simulink library "GAS"  (Simulink 8.5)
settings: Solver=ode45  StartTime=0.0  StopTime=10.0  RelTol=1e-3
undefined symbols (not defined in the file): COILOUTF, SIXOSEM_F_COILOUTF_MASTER, SIXOSEM_F_STAGE_MASTER
libraries: cdsEpicsOut x14, cdsFiltCtrl x4, cdsFilt x4, cdsTP x4, cdsEpicsIn x2, cdsEpicsBinIn x1, cdsFunctionCall x1, VIS_LIB x1
settings Model: Creator=controls  LastModifiedBy=controls

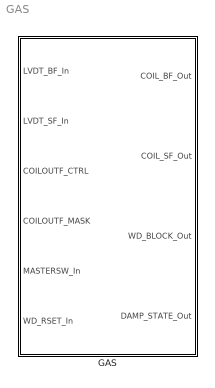
== system GAS ==
  GAS : Subsystem  Description=SIXOSEMSTAGE_FACE_MASTER  AncestorBlock=SIXOSEM_F_STAGE_MASTER/SIXOSEM_F_STAGE_MASTER

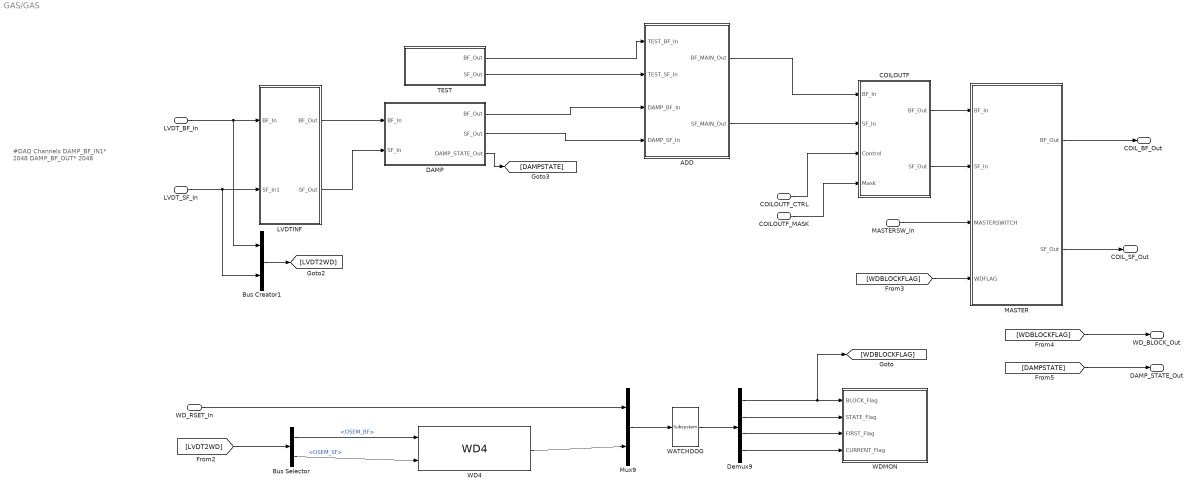
== system GAS/GAS ==
  note: #DAQ Channels
      | DAMP_BF_IN1* 2048
      | DAMP_BF_OUT* 2048
  LVDT_BF_In : Inport
  LVDT_SF_In : Inport  Port=2
  COILOUTF_CTRL : Inport  Port=3
  COILOUTF_MASK : Inport  Port=4
  MASTERSW_In : Inport  Port=5
  WD_RSET_In : Inport  Port=6
  ADD : Subsystem
  Bus Creator1 : BusCreator  Inputs='OSEM_BF','OSEM_SF'
  Bus Selector : BusSelector  OutputSignals=OSEM_BF,OSEM_SF
  COILOUTF : Subsystem  AncestorBlock=SIXOSEM_F_COILOUTF_MASTER/COILOUTF
  DAMP : Subsystem
  Demux9 : Demux
  LVDTINF : Subsystem
  MASTER : Subsystem
  Mux9 : Mux  Inputs=2
  TEST : Subsystem  AncestorBlock=SIXOSEM_F_STAGE_MASTER/SIXOSEM_F_STAGE_MASTER/TEST
  WATCHDOG : cdsFunctionCall/Subsystem  Tag=cdsFunctionCall  Description=inline OSEMWATCHDOG /opt/rtcds/userapps/release/vis/common/src/WATCHDOG.c
      settings: AttributesFormatString=%<Tag>\n%<Description>
  WD4 : VIS_LIB/WD4
  WDMON : Subsystem
  COIL_BF_Out : Outport
  COIL_SF_Out : Outport  Port=2
  WD_BLOCK_Out : Outport  Port=3
  DAMP_STATE_Out : Outport  Port=4
  wires:
  Bus Selector/1 -> WD4/1  "<OSEM_BF>"
  COILOUTF/1(BF_Out) -> MASTER/1(BF_In)
  ADD/1(BF_MAIN_Out) -> COILOUTF/1(BF_In)
  TEST/1(BF_Out) -> ADD/1(TEST_BF_In)
  LVDTINF/1(BF_Out) -> DAMP/1(BF_In)
  WATCHDOG/1 -> Demux9/1
  Mux9/1 -> WATCHDOG/1
  Demux9/4 -> WDMON/4(CURRENT_Flag)
  Demux9/3 -> WDMON/3(FIRST_Flag)
  Demux9/2 -> WDMON/2(STATE_Flag)
  Demux9/1 -> WDMON/1(BLOCK_Flag), [WDBLOCKFLAG]
  MASTER/1(BF_Out) -> COIL_BF_Out/1
  [LVDT2WD] -> Bus Selector/1
  Bus Creator1/1 -> [LVDT2WD]
  LVDT_BF_In/1 -> Bus Creator1/1, LVDTINF/1(BF_In)
  [WDBLOCKFLAG] -> MASTER/4(WDFLAG)
  [WDBLOCKFLAG] -> WD_BLOCK_Out/1
  DAMP/3(DAMP_STATE_Out) -> [DAMPSTATE]
  [DAMPSTATE] -> DAMP_STATE_Out/1
  MASTERSW_In/1 -> MASTER/3(MASTERSWITCH)
  COILOUTF_MASK/1 -> COILOUTF/4(Mask)
  COILOUTF_CTRL/1 -> COILOUTF/3(Control)
  WD4/1 -> Mux9/2
  WD_RSET_In/1 -> Mux9/1
  DAMP/1(BF_Out) -> ADD/3(DAMP_BF_In)
  LVDT_SF_In/1 -> Bus Creator1/2, LVDTINF/2(SF_In1)
  LVDTINF/2(SF_Out) -> DAMP/2(SF_In)
  TEST/2(SF_Out) -> ADD/2(TEST_SF_In)
  DAMP/2(SF_Out) -> ADD/4(DAMP_SF_In)
  ADD/2(SF_MAIN_Out) -> COILOUTF/2(SF_In)
  COILOUTF/2(SF_Out) -> MASTER/2(SF_In)
  MASTER/2(SF_Out) -> COIL_SF_Out/1
  Bus Selector/2 -> WD4/2  "<OSEM_SF>"

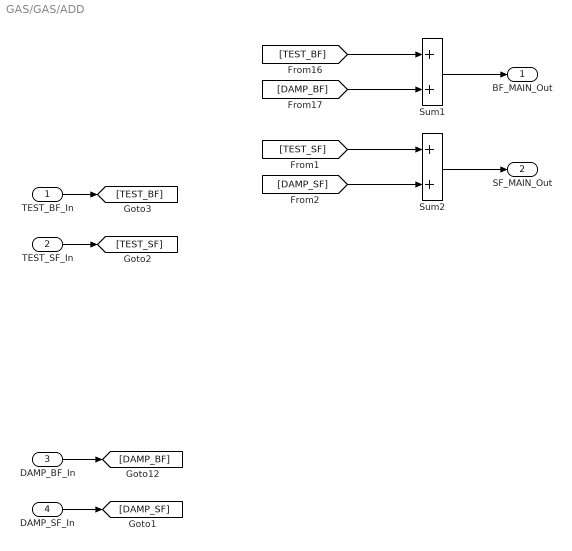
== system GAS/GAS/ADD ==
  TEST_BF_In : Inport
  TEST_SF_In : Inport  Port=2
  DAMP_BF_In : Inport  Port=3
  DAMP_SF_In : Inport  Port=4
  Sum1 : Sum
  Sum2 : Sum
  BF_MAIN_Out : Outport
  SF_MAIN_Out : Outport  Port=2
  wires:
  Sum1/1 -> BF_MAIN_Out/1
  TEST_BF_In/1 -> [TEST_BF]
  DAMP_BF_In/1 -> [DAMP_BF]
  [TEST_BF] -> Sum1/1
  [DAMP_BF] -> Sum1/2
  TEST_SF_In/1 -> [TEST_SF]
  DAMP_SF_In/1 -> [DAMP_SF]
  Sum2/1 -> SF_MAIN_Out/1
  [TEST_SF] -> Sum2/1
  [DAMP_SF] -> Sum2/2

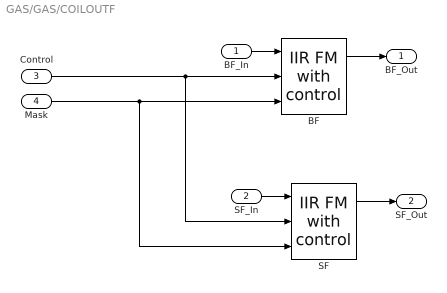
== system GAS/GAS/COILOUTF ==
  BF_In : Inport
  SF_In : Inport  Port=2
  Control : Inport  Port=3
  Mask : Inport  Port=4
  BF : cdsFiltCtrl/IIR FM with control  Tag=cdsFiltCtrl  Description=|
      | cdsFiltCntrl is the standard IIR filter module (exactly the same as cdsFilt) but with added control data output 'Ctrl'. Filter module digital signal output appears on the first output, which is called 'Val'. 'Ctrl' output has a bit pattern encoding the state of filter's on/off switches (FM1 through FM10). The bit values are:
      |                                                                                                                                                                                                                                                                                                                                       
      | module 	hex	dec                                                                                                                                                                                                                                                                                                                       
      | -----------------------                                                                                                                                                                                                                                                                                                               
      | FM1	0x20                    32                                                                                                                                                                                                                                                                                                        
      | FM2	0x80                     128                                                                                                                                                                                                                                                                                                      
      | FM3	0x200                   512                                                                                                                                                                                                                                                                                                       
      | FM4	0x800                   2048                                                                                                                                                                                                                                                                                                      
      | FM5	0x2000                 8192                                                                                                                                                                                                                                                                                                       
      | FM6	0x8000                 32768                                                                                                                                                                                                                                                                                                      
      | FM7	0x20000                131072                                                                                                                                                                                                                                                                                                     
      | FM8	0x80000                 524288                                                                                                                                                                                                                                                                                                    
      | FM9	0x200000               2097152                                                                                                                                                                                                                                                                                                    
      | FM10	0x800000               8388608                                                                                                                                                                                                                                                                                                   
      |                                                                                                                                                                                                                                                                                                                                       
      | This bit data can be used to drive some other switches or it can be output using a binary I/O module.
      settings: AttributesFormatString=%<Tag>
  SF : cdsFiltCtrl/IIR FM with control  Tag=cdsFiltCtrl  Description=|
      | cdsFiltCntrl is the standard IIR filter module (exactly the same as cdsFilt) but with added control data output 'Ctrl'. Filter module digital signal output appears on the first output, which is called 'Val'. 'Ctrl' output has a bit pattern encoding the state of filter's on/off switches (FM1 through FM10). The bit values are:
      |                                                                                                                                                                                                                                                                                                                                       
      | module 	hex	dec                                                                                                                                                                                                                                                                                                                       
      | -----------------------                                                                                                                                                                                                                                                                                                               
      | FM1	0x20                    32                                                                                                                                                                                                                                                                                                        
      | FM2	0x80                     128                                                                                                                                                                                                                                                                                                      
      | FM3	0x200                   512                                                                                                                                                                                                                                                                                                       
      | FM4	0x800                   2048                                                                                                                                                                                                                                                                                                      
      | FM5	0x2000                 8192                                                                                                                                                                                                                                                                                                       
      | FM6	0x8000                 32768                                                                                                                                                                                                                                                                                                      
      | FM7	0x20000                131072                                                                                                                                                                                                                                                                                                     
      | FM8	0x80000                 524288                                                                                                                                                                                                                                                                                                    
      | FM9	0x200000               2097152                                                                                                                                                                                                                                                                                                    
      | FM10	0x800000               8388608                                                                                                                                                                                                                                                                                                   
      |                                                                                                                                                                                                                                                                                                                                       
      | This bit data can be used to drive some other switches or it can be output using a binary I/O module.
      settings: AttributesFormatString=%<Tag>
  BF_Out : Outport
  SF_Out : Outport  Port=2
  wires:
  BF_In/1 -> BF/1
  BF/1 -> BF_Out/1
  Control/1 -> SF/2, BF/2
  Mask/1 -> SF/3, BF/3
  SF_In/1 -> SF/1
  SF/1 -> SF_Out/1

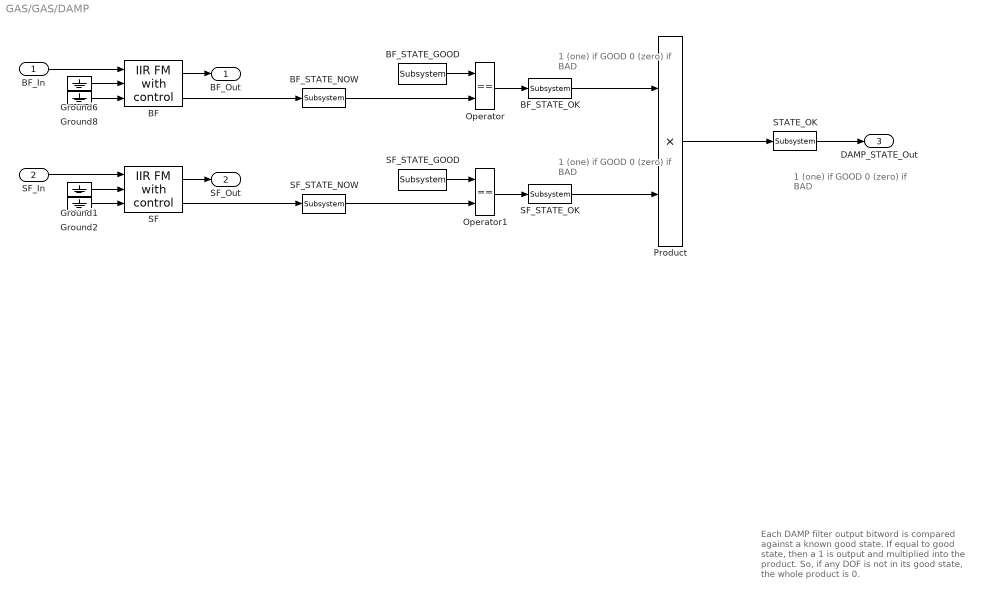
== system GAS/GAS/DAMP ==
  note: Each DAMP filter output bitword is
      | compared against a known good state.
      | If equal to good state, then a 1 is output
      | and multiplied into the product. So, if any DOF
      | is not in its good state, the whole product is 0.
  note: 1 (one) if GOOD
      | 0 (zero) if BAD
  note: 1 (one) if GOOD
      | 0 (zero) if BAD
  note: 1 (one) if GOOD
      | 0 (zero) if BAD
  BF_In : Inport
  SF_In : Inport  Port=2
  BF : cdsFiltCtrl/IIR FM with control  Tag=cdsFiltCtrl  Description=|
      | cdsFiltCntrl is the standard IIR filter module (exactly the same as cdsFilt) but with added control data output 'Ctrl'. Filter module digital signal output appears on the first output, which is called 'Val'. 'Ctrl' output has a bit pattern encoding the state of filter's on/off switches (FM1 through FM10). The bit values are:
      |                                                                                                                                                                                                                                                                                                                                       
      | module 	hex	dec                                                                                                                                                                                                                                                                                                                       
      | -----------------------                                                                                                                                                                                                                                                                                                               
      | FM1	0x20                    32                                                                                                                                                                                                                                                                                                        
      | FM2	0x80                     128                                                                                                                                                                                                                                                                                                      
      | FM3	0x200                   512                                                                                                                                                                                                                                                                                                       
      | FM4	0x800                   2048                                                                                                                                                                                                                                                                                                      
      | FM5	0x2000                 8192                                                                                                                                                                                                                                                                                                       
      | FM6	0x8000                 32768                                                                                                                                                                                                                                                                                                      
      | FM7	0x20000                131072                                                                                                                                                                                                                                                                                                     
      | FM8	0x80000                 524288                                                                                                                                                                                                                                                                                                    
      | FM9	0x200000               2097152                                                                                                                                                                                                                                                                                                    
      | FM10	0x800000               8388608                                                                                                                                                                                                                                                                                                   
      |                                                                                                                                                                                                                                                                                                                                       
      | This bit data can be used to drive some other switches or it can be output using a binary I/O module.
      settings: AttributesFormatString=%<Tag>
  BF_STATE_GOOD : cdsEpicsIn/Subsystem  Tag=cdsEpicsIn  Description=|
      | Purpose:                                                                              
      | Create an EPICS input channel connection to the FE realtime controls.                 
      |                                                                                       
      | Operation:                                                                            
      | Outputs value from an EPICS ai record. Value is floating point with a precision of 3..
      |                                                                                       
      | Usage:                                                                                
      | Name the part with the desired EPICS channel name.
      settings: AttributesFormatString=%<Tag>
  BF_STATE_NOW : cdsEpicsOut/Subsystem  Tag=cdsEpicsOutput  Description=|
      | Purpose:                                          
      | Output a FE signal to an EPICS channel.           
      |                                                   
      | Operation:                                        
      | Takes input value and passes it to EPICS record.  
      |                                                   
      | Usage:                                            
      | Name the part with the desired EPICS rrecord name.
      settings: AttributesFormatString=%<Tag>
  BF_STATE_OK : cdsEpicsOut/Subsystem  Tag=cdsEpicsOutput  Description=|
      | Purpose:                                          
      | Output a FE signal to an EPICS channel.           
      |                                                   
      | Operation:                                        
      | Takes input value and passes it to EPICS record.  
      |                                                   
      | Usage:                                            
      | Name the part with the desired EPICS rrecord name.
      settings: AttributesFormatString=%<Tag>
  Ground{1..2,6,8} (4 alike) : Ground
  Operator : RelationalOperator  Operator===  OutDataTypeStr=boolean
  Operator1 : RelationalOperator  Operator===  OutDataTypeStr=boolean
  Product : Product  RndMeth=Zero
  SF : cdsFiltCtrl/IIR FM with control  Tag=cdsFiltCtrl  Description=|
      | cdsFiltCntrl is the standard IIR filter module (exactly the same as cdsFilt) but with added control data output 'Ctrl'. Filter module digital signal output appears on the first output, which is called 'Val'. 'Ctrl' output has a bit pattern encoding the state of filter's on/off switches (FM1 through FM10). The bit values are:
      |                                                                                                                                                                                                                                                                                                                                       
      | module 	hex	dec                                                                                                                                                                                                                                                                                                                       
      | -----------------------                                                                                                                                                                                                                                                                                                               
      | FM1	0x20                    32                                                                                                                                                                                                                                                                                                        
      | FM2	0x80                     128                                                                                                                                                                                                                                                                                                      
      | FM3	0x200                   512                                                                                                                                                                                                                                                                                                       
      | FM4	0x800                   2048                                                                                                                                                                                                                                                                                                      
      | FM5	0x2000                 8192                                                                                                                                                                                                                                                                                                       
      | FM6	0x8000                 32768                                                                                                                                                                                                                                                                                                      
      | FM7	0x20000                131072                                                                                                                                                                                                                                                                                                     
      | FM8	0x80000                 524288                                                                                                                                                                                                                                                                                                    
      | FM9	0x200000               2097152                                                                                                                                                                                                                                                                                                    
      | FM10	0x800000               8388608                                                                                                                                                                                                                                                                                                   
      |                                                                                                                                                                                                                                                                                                                                       
      | This bit data can be used to drive some other switches or it can be output using a binary I/O module.
      settings: AttributesFormatString=%<Tag>
  SF_STATE_GOOD : cdsEpicsIn/Subsystem  Tag=cdsEpicsIn  Description=|
      | Purpose:                                                                              
      | Create an EPICS input channel connection to the FE realtime controls.                 
      |                                                                                       
      | Operation:                                                                            
      | Outputs value from an EPICS ai record. Value is floating point with a precision of 3..
      |                                                                                       
      | Usage:                                                                                
      | Name the part with the desired EPICS channel name.
      settings: AttributesFormatString=%<Tag>
  SF_STATE_NOW : cdsEpicsOut/Subsystem  Tag=cdsEpicsOutput  Description=|
      | Purpose:                                          
      | Output a FE signal to an EPICS channel.           
      |                                                   
      | Operation:                                        
      | Takes input value and passes it to EPICS record.  
      |                                                   
      | Usage:                                            
      | Name the part with the desired EPICS rrecord name.
      settings: AttributesFormatString=%<Tag>
  SF_STATE_OK : cdsEpicsOut/Subsystem  Tag=cdsEpicsOutput  Description=|
      | Purpose:                                          
      | Output a FE signal to an EPICS channel.           
      |                                                   
      | Operation:                                        
      | Takes input value and passes it to EPICS record.  
      |                                                   
      | Usage:                                            
      | Name the part with the desired EPICS rrecord name.
      settings: AttributesFormatString=%<Tag>
  STATE_OK : cdsEpicsOut/Subsystem  Tag=cdsEpicsOutput  Description=|
      | Purpose:                                          
      | Output a FE signal to an EPICS channel.           
      |                                                   
      | Operation:                                        
      | Takes input value and passes it to EPICS record.  
      |                                                   
      | Usage:                                            
      | Name the part with the desired EPICS rrecord name.
      settings: AttributesFormatString=%<Tag>
  BF_Out : Outport
  SF_Out : Outport  Port=2
  DAMP_STATE_Out : Outport  Port=3
  wires:
  Ground6/1 -> BF/2
  BF_In/1 -> BF/1
  BF/1 -> BF_Out/1
  BF_STATE_GOOD/1 -> Operator/1
  BF/2 -> BF_STATE_NOW/1
  Operator/1 -> BF_STATE_OK/1
  BF_STATE_NOW/1 -> Operator/2
  STATE_OK/1 -> DAMP_STATE_Out/1
  Ground8/1 -> BF/3
  Ground1/1 -> SF/2
  SF_In/1 -> SF/1
  SF/1 -> SF_Out/1
  SF_STATE_GOOD/1 -> Operator1/1
  SF/2 -> SF_STATE_NOW/1
  Operator1/1 -> SF_STATE_OK/1
  SF_STATE_NOW/1 -> Operator1/2
  Ground2/1 -> SF/3
  SF_STATE_OK/1 -> Product/2
  BF_STATE_OK/1 -> Product/1
  Product/1 -> STATE_OK/1

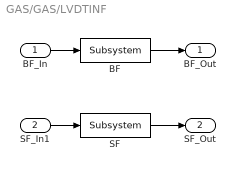
== system GAS/GAS/LVDTINF ==
  BF_In : Inport
  SF_In1 : Inport  Port=2
  BF : cdsFilt/Subsystem  Tag=cdsFilt  Description=|
      | Purpose:                                                                                                                                                                                                                                  
      | Standard CDS IIR filter module.                                                                                                                                                                                                           
      |                                                                                                                                                                                                                                           
      | Operation:                                                                                                                                                                                                                                
      | Consists of 10 second order section IIR filters, plus a ramped gain stage. In FE code, also provides pre-defined test points and excitation channel inputs. The filter coefficients are defined in the LIGO system using the 'foton' tool.
      |                                                                                                                                                                                                                                           
      | Usage:                                                                                                                                                                                                                                    
      | Name the part with the desired filter module name.
      settings: AttributesFormatString=%<Tag>
  SF : cdsFilt/Subsystem  Tag=cdsFilt  Description=|
      | Purpose:                                                                                                                                                                                                                                  
      | Standard CDS IIR filter module.                                                                                                                                                                                                           
      |                                                                                                                                                                                                                                           
      | Operation:                                                                                                                                                                                                                                
      | Consists of 10 second order section IIR filters, plus a ramped gain stage. In FE code, also provides pre-defined test points and excitation channel inputs. The filter coefficients are defined in the LIGO system using the 'foton' tool.
      |                                                                                                                                                                                                                                           
      | Usage:                                                                                                                                                                                                                                    
      | Name the part with the desired filter module name.
      settings: AttributesFormatString=%<Tag>
  BF_Out : Outport
  SF_Out : Outport  Port=2
  wires:
  BF_In/1 -> BF/1
  BF/1 -> BF_Out/1
  SF_In1/1 -> SF/1
  SF/1 -> SF_Out/1

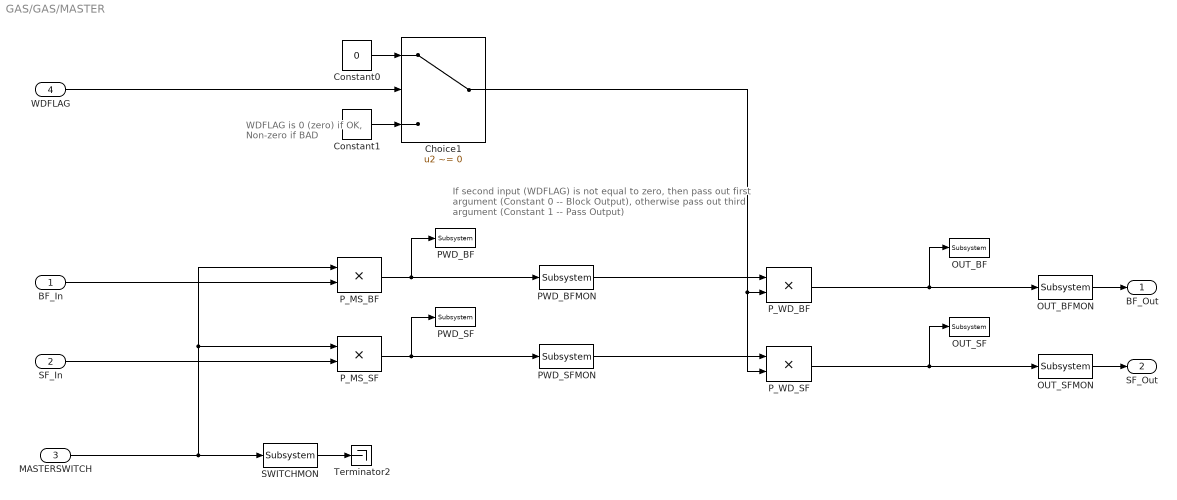
== system GAS/GAS/MASTER ==
  note: WDFLAG is 0 (zero) if OK,
      | Non-zero if BAD
  note: If second input (WDFLAG) is not equal to zero,
      | then pass out first argument (Constant 0 -- Block Output),
      | otherwise pass out third argument (Constant 1 -- Pass Output)
  BF_In : Inport
  SF_In : Inport  Port=2
  MASTERSWITCH : Inport  Port=3
  WDFLAG : Inport  Port=4
  Choice1 : Switch  Criteria=u2 ~= 0  Threshold=0.5
  Constant0 : Constant  Value=0
  Constant1 : Constant
  OUT_BF : cdsTP/Subsystem  Tag=Test Point
      settings: AttributesFormatString=%<Tag>
  OUT_BFMON : cdsEpicsOut/Subsystem  Tag=cdsEpicsOutput  Description=|
      | Purpose:                                          
      | Output a FE signal to an EPICS channel.           
      |                                                   
      | Operation:                                        
      | Takes input value and passes it to EPICS record.  
      |                                                   
      | Usage:                                            
      | Name the part with the desired EPICS rrecord name.
      settings: AttributesFormatString=%<Tag>
  OUT_SF : cdsTP/Subsystem  Tag=Test Point
      settings: AttributesFormatString=%<Tag>
  OUT_SFMON : cdsEpicsOut/Subsystem  Tag=cdsEpicsOutput  Description=|
      | Purpose:                                          
      | Output a FE signal to an EPICS channel.           
      |                                                   
      | Operation:                                        
      | Takes input value and passes it to EPICS record.  
      |                                                   
      | Usage:                                            
      | Name the part with the desired EPICS rrecord name.
      settings: AttributesFormatString=%<Tag>
  PWD_BF : cdsTP/Subsystem  Tag=Test Point
      settings: AttributesFormatString=%<Tag>
  PWD_BFMON : cdsEpicsOut/Subsystem  Tag=cdsEpicsOutput  Description=|
      | Purpose:                                          
      | Output a FE signal to an EPICS channel.           
      |                                                   
      | Operation:                                        
      | Takes input value and passes it to EPICS record.  
      |                                                   
      | Usage:                                            
      | Name the part with the desired EPICS rrecord name.
      settings: AttributesFormatString=%<Tag>
  PWD_SF : cdsTP/Subsystem  Tag=Test Point
      settings: AttributesFormatString=%<Tag>
  PWD_SFMON : cdsEpicsOut/Subsystem  Tag=cdsEpicsOutput  Description=|
      | Purpose:                                          
      | Output a FE signal to an EPICS channel.           
      |                                                   
      | Operation:                                        
      | Takes input value and passes it to EPICS record.  
      |                                                   
      | Usage:                                            
      | Name the part with the desired EPICS rrecord name.
      settings: AttributesFormatString=%<Tag>
  P_MS_BF : Product  RndMeth=Zero
  P_MS_SF : Product  RndMeth=Zero
  P_WD_BF : Product  RndMeth=Zero
  P_WD_SF : Product  RndMeth=Zero
  SWITCHMON : cdsEpicsOut/Subsystem  Tag=cdsEpicsOutput  Description=|
      | Purpose:                                          
      | Output a FE signal to an EPICS channel.           
      |                                                   
      | Operation:                                        
      | Takes input value and passes it to EPICS record.  
      |                                                   
      | Usage:                                            
      | Name the part with the desired EPICS rrecord name.
      settings: AttributesFormatString=%<Tag>
  Terminator2 : Terminator
  BF_Out : Outport
  SF_Out : Outport  Port=2
  wires:
  Choice1/1 -> P_WD_SF/2, P_WD_BF/2
  PWD_BFMON/1 -> P_WD_BF/1
  WDFLAG/1 -> Choice1/2
  Constant0/1 -> Choice1/1
  Constant1/1 -> Choice1/3
  P_WD_BF/1 -> OUT_BF/1, OUT_BFMON/1
  P_MS_BF/1 -> PWD_BFMON/1, PWD_BF/1
  OUT_BFMON/1 -> BF_Out/1
  MASTERSWITCH/1 -> P_MS_SF/1, P_MS_BF/1, SWITCHMON/1
  BF_In/1 -> P_MS_BF/2
  SWITCHMON/1 -> Terminator2/1
  PWD_SFMON/1 -> P_WD_SF/1
  P_WD_SF/1 -> OUT_SF/1, OUT_SFMON/1
  P_MS_SF/1 -> PWD_SFMON/1, PWD_SF/1
  OUT_SFMON/1 -> SF_Out/1
  SF_In/1 -> P_MS_SF/2

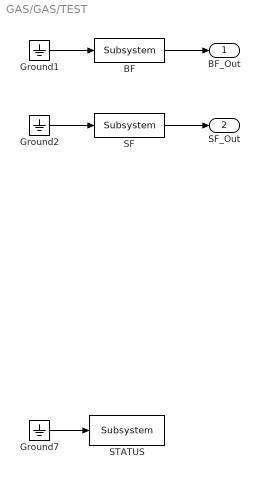
== system GAS/GAS/TEST ==
  BF : cdsFilt/Subsystem  Tag=cdsFilt  Description=|
      | Purpose:                                                                                                                                                                                                                                  
      | Standard CDS IIR filter module.                                                                                                                                                                                                           
      |                                                                                                                                                                                                                                           
      | Operation:                                                                                                                                                                                                                                
      | Consists of 10 second order section IIR filters, plus a ramped gain stage. In FE code, also provides pre-defined test points and excitation channel inputs. The filter coefficients are defined in the LIGO system using the 'foton' tool.
      |                                                                                                                                                                                                                                           
      | Usage:                                                                                                                                                                                                                                    
      | Name the part with the desired filter module name.
      settings: AttributesFormatString=%<Tag>
  Ground1 : Ground
  Ground2 : Ground
  Ground7 : Ground
  SF : cdsFilt/Subsystem  Tag=cdsFilt  Description=|
      | Purpose:                                                                                                                                                                                                                                  
      | Standard CDS IIR filter module.                                                                                                                                                                                                           
      |                                                                                                                                                                                                                                           
      | Operation:                                                                                                                                                                                                                                
      | Consists of 10 second order section IIR filters, plus a ramped gain stage. In FE code, also provides pre-defined test points and excitation channel inputs. The filter coefficients are defined in the LIGO system using the 'foton' tool.
      |                                                                                                                                                                                                                                           
      | Usage:                                                                                                                                                                                                                                    
      | Name the part with the desired filter module name.
      settings: AttributesFormatString=%<Tag>
  STATUS : cdsEpicsBinIn/Subsystem  Tag=cdsEpicsBinIn  Description=|
      | Purpose:                                                                            
      | Create an EPICS binary (0 or 1) input channel to the FE realtime controls.          
      |                                                                                     
      | Operation:                                                                          
      | Outputs value from an EPICS ai record. Value is binary input (bi Epics record type).
      |                                                                                     
      | Usage:                                                                              
      | Name the part with the desired EPICS channel name.
      settings: AttributesFormatString=%<Tag>
  BF_Out : Outport
  SF_Out : Outport  Port=2
  wires:
  Ground7/1 -> STATUS/1
  Ground1/1 -> BF/1
  BF/1 -> BF_Out/1
  Ground2/1 -> SF/1
  SF/1 -> SF_Out/1

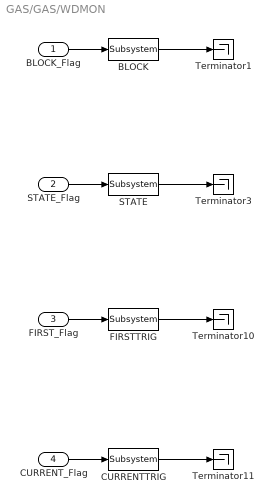
== system GAS/GAS/WDMON ==
  BLOCK_Flag : Inport
  STATE_Flag : Inport  Port=2
  FIRST_Flag : Inport  Port=3
  CURRENT_Flag : Inport  Port=4
  BLOCK : cdsEpicsOut/Subsystem  Tag=cdsEpicsOutput  Description="field(PREC,\"3\")"
      settings: AttributesFormatString=%<Tag>
  CURRENTTRIG : cdsEpicsOut/Subsystem  Tag=cdsEpicsOutput  Description="field(PREC,\"3\")"
      settings: AttributesFormatString=%<Tag>
  FIRSTTRIG : cdsEpicsOut/Subsystem  Tag=cdsEpicsOutput  Description="field(PREC,\"3\")"
      settings: AttributesFormatString=%<Tag>
  STATE : cdsEpicsOut/Subsystem  Tag=cdsEpicsOutput  Description="field(PREC,\"3\")"
      settings: AttributesFormatString=%<Tag>
  Terminator{1,3,10..11} (4 alike) : Terminator
  wires:
  STATE/1 -> Terminator3/1
  BLOCK/1 -> Terminator1/1
  BLOCK_Flag/1 -> BLOCK/1
  FIRSTTRIG/1 -> Terminator10/1
  CURRENTTRIG/1 -> Terminator11/1
  CURRENT_Flag/1 -> CURRENTTRIG/1
  FIRST_Flag/1 -> FIRSTTRIG/1
  STATE_Flag/1 -> STATE/1
